simulink model "filter_IIR1"  (Simulink 7.9)
settings: Solver=ode3  StartTime=0.0  StopTime=20  FixedStep=0.125e-3  RelTol=1e-3
libraries: dspstat3 x1, simulink x1
settings Model: Creator=asus  LastModifiedBy=asus

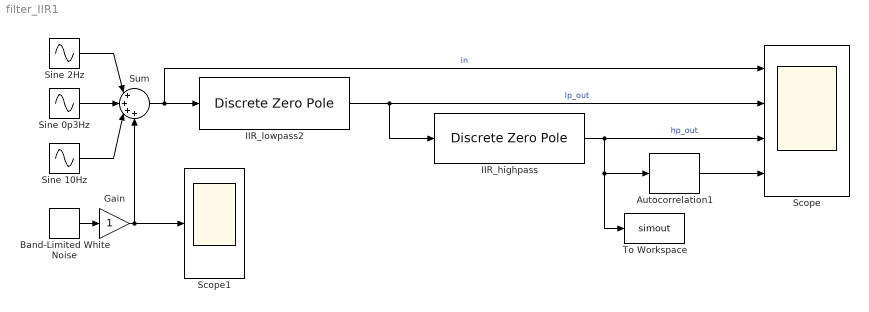
== system filter_IIR1 ==
  Autocorrelation1 : dspstat3/Autocorrelation  AllPositiveLags=on  maxlag=1  bias=Unbiased  domain=Time  outputDataTypeStr=Inherit: Same as accumulator  outputLastDataTypeStr=Inherit: Same as accumulator  outputMin=[]  outputMax=[]  roundingMode=Floor  overflowMode=off
  Band-Limited White Noise : simulink/Sources/Band-Limited White Noise  Cov=[1.25e-7]  Ts=0.125e-3  seed=[23341]
  Gain : Gain
  IIR_highpass : DiscreteZeroPole  Zeros=ones(1,20)  Poles=4095/4096*ones(1,20)  Gain=(4095/4096)^15  SampleTime=0.125e-3
  IIR_lowpass2 : DiscreteZeroPole  Zeros=zeros(1,5)  Poles=255/256*ones(1,5)  Gain=(1-255/256)^5*2^3  SampleTime=0.125e-3
  Scope : Scope  NumInputPorts=4
      settings: ShowLegends=on  TimeRange=20  YMin=0.98~-2~-2.5~-5  YMax=1.04~2~2.5~5  MaxDataPoints=65536  SampleInput=on  SampleTime=0.125e-3
  Scope1 : Scope
      settings: ShowLegends=on  TimeRange=19  YMin=0.98  YMax=1.04  MaxDataPoints=65536  SampleInput=on  SampleTime=0.125e-3
  Sine 0p3Hz : Sin  Amplitude=0  Frequency=0.3*2*pi  SampleTime=0.125e-3
  Sine 10Hz : Sin  Amplitude=0  Frequency=10*2*pi  SampleTime=0.125e-3
  Sine 2Hz : Sin  Amplitude=20e-3  Frequency=2*2*pi  SampleTime=0.125e-3
  Sum : Sum  Inputs=|++++  SampleTime=0.125e-3
  To Workspace : ToWorkspace  VariableName=simout  SampleTime=0.125e-3
  wires:
  Sine 2Hz/1 -> Sum/1
  Sum/1 -> Scope/1, IIR_lowpass2/1  "in"
  Sine 0p3Hz/1 -> Sum/2
  Sine 10Hz/1 -> Sum/3
  Band-Limited White Noise/1 -> Gain/1
  IIR_lowpass2/1 -> Scope/2, IIR_highpass/1  "lp_out"
  IIR_highpass/1 -> Scope/3, To Workspace/1, Autocorrelation1/1  "hp_out"
  Gain/1 -> Sum/4, Scope1/1
  Autocorrelation1/1 -> Scope/4
